simulink model "lab6_exp2_2019a"  (R2019a)
settings: Solver=FixedStepAuto  StartTime=0.0  StopTime=inf  RelTol=1e-3  EnableMultiTasking=on
undefined symbols (not defined in the file): DiscIntNeverNeededParam
libraries: arduinolib x2, simulink x1
settings Model: ExtModeTrigDuration=2  Creator=student  LastModifiedBy=student
settings OptimizationCC: EnhancedBackFolding=on  PassReuseOutputArgsAs=Individual arguments  MaxStackSize=64  OptimizeBlockOrder=speed  DifferentSizesBufferReuse=on  OptimizationCustomize=off
settings DebuggingCC: ParameterTunabilityLossMsg=error
settings HardwareCC: ProdBitPerInt=16  ProdBitPerPointer=16  ProdBitPerSizeT=16  ProdBitPerPtrDiffT=16  ProdLargestAtomicFloat=None  ProdWordSize=8  ProdHWDeviceType=Atmel->AVR
settings SFSimCC: MATLABDynamicMemAlloc=off
settings RTWCC: SystemTargetFile=ert.tlc  HardwareBoard=Arduino Uno  TLCOptions=-aInlineSetEventsForThisBaseRateFcn=TLC_FALSE -aSuppressMultiTaskScheduler=TLC_FALSE -aRateBasedStepFcn=1  TemplateMakefile=ert_default_tmf  GenerateReport=on  Toolchain=Arduino AVR  BuildConfiguration=Faster Runs  IncludeHyperlinkInReport=on  LaunchReport=on  GenerateTraceInfo=on  GenerateTraceReport=on  GenerateTraceReportSl=on  GenerateTraceReportSf=on  GenerateTraceReportEml=on
settings CodeAppCC: ForceParamTrailComments=on  IgnoreCustomStorageClasses=off  OperatorAnnotations=on  SimulinkDataObjDesc=on  SFDataObjDesc=on  InsertBlockDesc=on
settings ERTTargetCC: SupportContinuousTime=on  SupportVariableSizeSignals=on  ExtModeStaticAllocSize=250

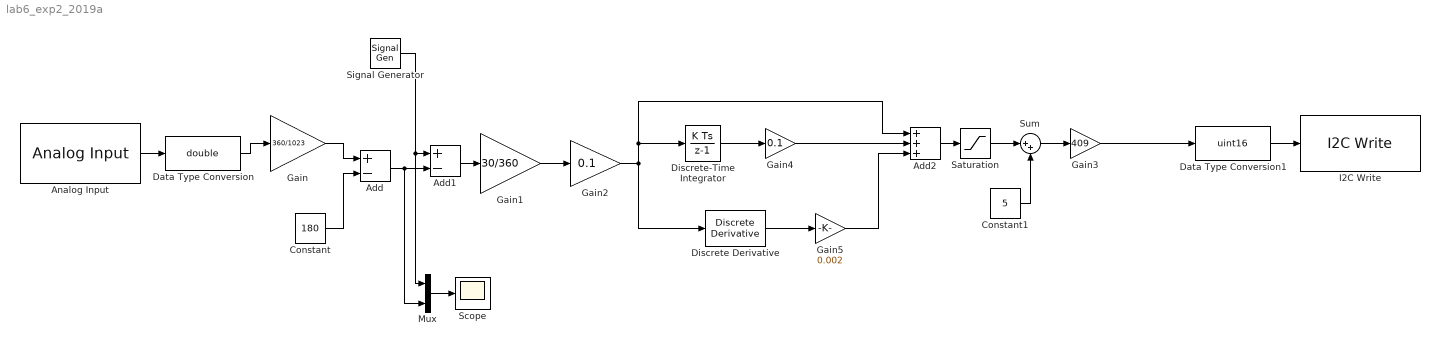
== system lab6_exp2_2019a ==
  Add : Sum  Inputs=+-
  Add1 : Sum  Inputs=+-
  Add2 : Sum  Inputs=+++
  Analog Input : arduinolib/Analog Input  pinNumber=1  ReadResultsOnly=off  ConversionTriggerSource=Software  ExternalTriggerType=uint32(0)  OutputDataType=uint16  EnableConversionCompleteNotify=off  EnableOuputStatus=off  SampleTime=0.02  blockPlatform=arduino
  Constant : Constant  Value=180
  Constant1 : Constant  Value=5
  Data Type Conversion : DataTypeConversion  OutDataTypeStr=double
  Data Type Conversion1 : DataTypeConversion  OutDataTypeStr=uint16
  Discrete Derivative : simulink/Discrete/Discrete Derivative  gainval=1.0  ICPrevScaledInput=0.0  OutMin=[]  OutMax=[]  OutDataType=fixdt(1, 16)  OutScaling=2^-10  DoSatur=off
  Discrete-Time Integrator : DiscreteIntegrator  gainval=1  SampleTime=-1  ICPrevOutput=DiscIntNeverNeededParam  ICPrevScaledInput=DiscIntNeverNeededParam
  Gain : Gain  Gain=360/1023
  Gain1 : Gain  Gain=30/360
  Gain2 : Gain  Gain=0.1
  Gain3 : Gain  Gain=409
  Gain4 : Gain  Gain=0.1
  Gain5 : Gain  Gain=0.002
  I2C Write : arduinolib/I2C Write  I2CModule=0  Mode=Master  SlaveAddress=hex2dec('60')  SlaveByteOrder=BigEndian  Direction=Transmitter  RegisterAddressMode=off  RegisterAddress=0  SlaveDataType=uint8  DataLength=1  NoAck=off  RepeatedStart=off  OutputStatus=off  blockPlatform=ARDUINO
      settings: SourceProductName=Simulink Support Package for Arduino Hardware  SourceProductBaseCode=ARDUINO
  Mux : Mux  Inputs=2
  Saturation : Saturate  UpperLimit=5  LowerLimit=-5
  Scope : Scope
  Signal Generator : SignalGenerator  WaveForm=square  Amplitude=45  Frequency=0.1
  Sum : Sum  Inputs=|++
  wires:
  Analog Input/1 -> Data Type Conversion/1
  Data Type Conversion1/1 -> I2C Write/1
  Data Type Conversion/1 -> Gain/1
  Gain/1 -> Add/1
  Constant/1 -> Add/2
  Gain1/1 -> Gain2/1
  Add1/1 -> Gain1/1
  Add/1 -> Mux/2, Add1/2
  Signal Generator/1 -> Mux/1, Add1/1
  Mux/1 -> Scope/1
  Gain2/1 -> Discrete Derivative/1, Discrete-Time Integrator/1, Add2/1
  Add2/1 -> Saturation/1
  Saturation/1 -> Sum/1
  Constant1/1 -> Sum/2
  Sum/1 -> Gain3/1
  Discrete-Time Integrator/1 -> Gain4/1
  Gain4/1 -> Add2/2
  Gain5/1 -> Add2/3
  Discrete Derivative/1 -> Gain5/1
  Gain3/1 -> Data Type Conversion1/1
